simulink model "Retro_Edo_1"  (Simulink 8.6)
settings: Solver=VariableStepAuto  SolverMode=SingleTasking  StartTime=0.0  StopTime=10.0  FixedStep=0.001  RelTol=1e-3
values from neighbouring files (symbols this model uses):
  A = [0 1 0 ... (first row only)    [COpt.m]    (also in Ob_Edo.m; Retro_Edo 2.m)
  b = [0; 0; 1]    [COpt.m]    (also in Ob_Edo.m; Retro_Edo 2.m)
  f1 = [1; 1; -1]    [Retro_Edo 2.m]
  Id = eye(3)    [COpt.m]    (also in Ob_Edo.m; Retro_Edo 2.m)
  T1 = inv(MO)*MOo    [Ob_Edo.m]
  vcero = zeros(3,1)    [COpt.m]    (also in Ob_Edo.m; Retro_Edo 2.m)
  x0 = [1; 0; 0]    [COpt.m]    (also in Ob_Edo.m; Retro_Edo 2.m)
settings Model: Creator=Tlakatl  LastModifiedBy=Tlayekanketl
settings DebuggingCC: SolverPrmCheckMsg=none  FcnCallInpInsideContextMsg=EnableAllAsWarning
settings ConfigComp: CovSFcnEnable=off

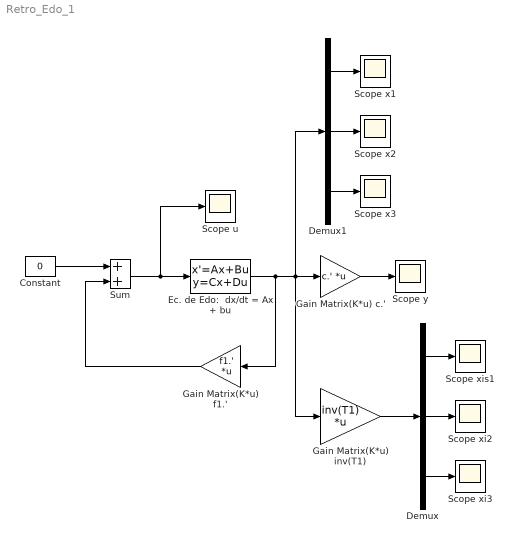
== system Retro_Edo_1 ==
  Constant : Constant  Value=0
  Demux : Demux  Outputs=3
  Demux1 : Demux  Outputs=3
  Ec. de Edo:  dx/dt = Ax + bu : StateSpace  A=A  B=b  C=Id  D=vcero  X0=x0
  Gain Matrix(K*u) c.' : Gain  Gain=c.'  Multiplication=Matrix(K*u)
  Gain Matrix(K*u) f1.' : Gain  Gain=f1.'  Multiplication=Matrix(K*u) (u vector)
  Gain Matrix(K*u) inv(T1) : Gain  Gain=inv(T1)  Multiplication=Matrix(K*u)
  Scope u : Scope
  Scope x1 : Scope
  Scope x2 : Scope
  Scope x3 : Scope
  Scope xi2 : Scope
  Scope xi3 : Scope
  Scope xis1 : Scope
  Scope y : Scope
  Sum : Sum
  wires:
  Sum/1 -> Ec. de Edo:  dx/dt = Ax + bu/1, Scope u/1
  Ec. de Edo:  dx/dt = Ax + bu/1 -> Gain Matrix(K*u) f1.'/1, Gain Matrix(K*u) c.'/1, Gain Matrix(K*u) inv(T1)/1, Demux1/1
  Gain Matrix(K*u) f1.'/1 -> Sum/2
  Constant/1 -> Sum/1
  Gain Matrix(K*u) c.'/1 -> Scope y/1
  Gain Matrix(K*u) inv(T1)/1 -> Demux/1
  Demux/3 -> Scope xi3/1
  Demux/2 -> Scope xi2/1
  Demux/1 -> Scope xis1/1
  Demux1/3 -> Scope x3/1
  Demux1/2 -> Scope x2/1
  Demux1/1 -> Scope x1/1
